simulink model "bluetooth_voice"  (Simulink 6.0)
settings: Solver=ode3  SolverMode=SingleTasking  StartTime=0.0  StopTime=2.7  RelTol=1e-3
PreLoadFcn:
  | bluetooth_init;
PostLoadFcn:
  | bluetooth_cb
values from neighbouring files (symbols this model uses):
  Access_Code = zeros(72,1); Access_Code(1:2:72)=1    [bluetooth_init.m]
  ARQ = [1]    [bluetooth_init.m]
  awgn_802_seed = randseed(3)    [bluetooth_init.m]
  awgn_channel_seed = randseed(2)    [bluetooth_init.m]
  data_seed = randseed(5)    [bluetooth_init.m]
  Flow_Control = [1]    [bluetooth_init.m]
  HV_Type = 3    [bluetooth_cb.m]
  Input_Fs = 8000    [bluetooth_init.m]
  One_Zero_Payload = zeros(240,1)    [bluetooth_init.m]
  Packet_Type = [1 0 1 0]'    [bluetooth_init.m]
  rate_802_seed = randseed(4)    [bluetooth_init.m]
  Sequence = [1]    [bluetooth_init.m]
  Slave_Address = [1 0 1]'    [bluetooth_init.m]
  Slot_Ts = (1/1600)    (= 0.000625)    [bluetooth_cb.m]
undefined symbols (not defined in the file or in its folder): figposition, Fs, jet, Num_Slots_Rate, slcm, Slot_Enable_Phase, Tx_Ts
libraries: commblkcod2 x48, dspsrcs4 x22, dspsigops x19, simulink x15, dspbuff3 x8, dspindex x7, dspsigattribs x6, dspmtrx3 x5, dsparch4 x4, commdigbbndfm2 x4, bluetooth_lib x4, dspsnks4 x4
(part 2 of 2)

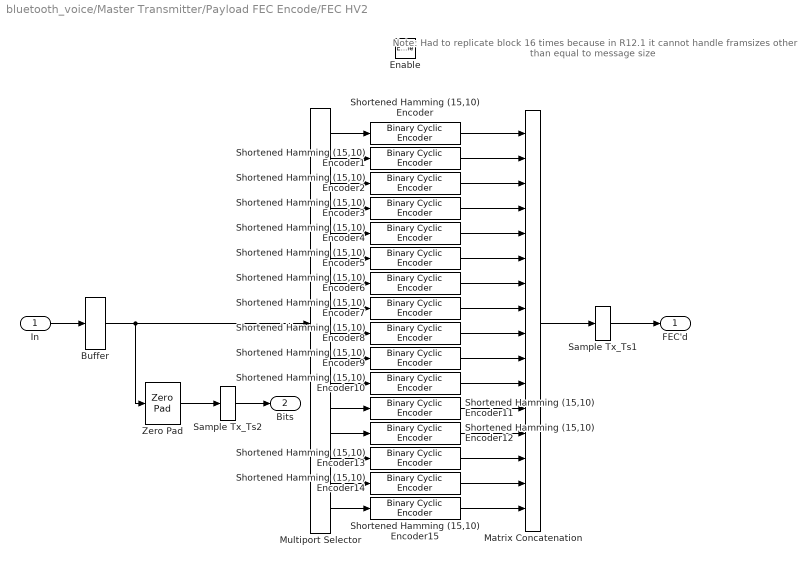
== system bluetooth_voice/Master Transmitter/Payload FEC Encode/FEC HV2 ==
  note: Note: Had to replicate block 16 times
      | because in R12.1 it cannot handle framsizes
      | other than equal to message size
  In : Inport  LatchInput=off
  Enable : EnablePort
  Buffer : dspbuff3/Buffer  N=160  V=0  ic=0
  Matrix Concatenation : simulink/Math Operations/Matrix Concatenation  numInports=16  catMethod=Vertical
  Multiport Selector : dspindex/Multiport Selector  rowsOrCols=Rows  idxCellArray={ 1:10, 11:20,21:30,31:40,41:50,51:60,61:70,71:80,81:90,91:100,101:110,111:120,121:130,131:140,141:150,151:160}  idxErrMode=Clip Index
  Sample Tx_Ts1 : ZeroOrderHold  SampleTime=Slot_Ts
  Sample Tx_Ts2 : ZeroOrderHold  SampleTime=Slot_Ts
  Shortened Hamming (15,10) Encoder{,1..15} (16 alike) : commblkcod2/Binary Cyclic Encoder  n=15  p=[1 1 0 1 0 1]
  Zero Pad : dspsigops/Zero Pad  padSigAt=End  zpadAlong=Columns  padNumOutRowsSpecMethod=User-specified  numOutRows=240  padNumOutColsSpecMethod=User-specified  numOutCols=1  trunc_flag=None
  FEC'd : Outport
  Bits : Outport  Port=2
  wires:
  In/1 -> Buffer/1
  Buffer/1 -> Multiport Selector/1, Zero Pad/1
  Multiport Selector/1 -> Shortened Hamming (15,10) Encoder/1
  Multiport Selector/2 -> Shortened Hamming (15,10) Encoder1/1
  Multiport Selector/3 -> Shortened Hamming (15,10) Encoder2/1
  Multiport Selector/4 -> Shortened Hamming (15,10) Encoder3/1
  Multiport Selector/5 -> Shortened Hamming (15,10) Encoder4/1
  Multiport Selector/6 -> Shortened Hamming (15,10) Encoder5/1
  Multiport Selector/7 -> Shortened Hamming (15,10) Encoder6/1
  Multiport Selector/8 -> Shortened Hamming (15,10) Encoder7/1
  Multiport Selector/9 -> Shortened Hamming (15,10) Encoder8/1
  Multiport Selector/10 -> Shortened Hamming (15,10) Encoder9/1
  Multiport Selector/11 -> Shortened Hamming (15,10) Encoder10/1
  Multiport Selector/12 -> Shortened Hamming (15,10) Encoder11/1
  Multiport Selector/13 -> Shortened Hamming (15,10) Encoder12/1
  Multiport Selector/14 -> Shortened Hamming (15,10) Encoder13/1
  Multiport Selector/15 -> Shortened Hamming (15,10) Encoder14/1
  Multiport Selector/16 -> Shortened Hamming (15,10) Encoder15/1
  Shortened Hamming (15,10) Encoder/1 -> Matrix Concatenation/1
  Shortened Hamming (15,10) Encoder1/1 -> Matrix Concatenation/2
  Shortened Hamming (15,10) Encoder2/1 -> Matrix Concatenation/3
  Shortened Hamming (15,10) Encoder3/1 -> Matrix Concatenation/4
  Shortened Hamming (15,10) Encoder4/1 -> Matrix Concatenation/5
  Shortened Hamming (15,10) Encoder5/1 -> Matrix Concatenation/6
  Shortened Hamming (15,10) Encoder6/1 -> Matrix Concatenation/7
  Shortened Hamming (15,10) Encoder7/1 -> Matrix Concatenation/8
  Shortened Hamming (15,10) Encoder8/1 -> Matrix Concatenation/9
  Shortened Hamming (15,10) Encoder9/1 -> Matrix Concatenation/10
  Shortened Hamming (15,10) Encoder10/1 -> Matrix Concatenation/11
  Shortened Hamming (15,10) Encoder11/1 -> Matrix Concatenation/12
  Shortened Hamming (15,10) Encoder12/1 -> Matrix Concatenation/13
  Shortened Hamming (15,10) Encoder13/1 -> Matrix Concatenation/14
  Shortened Hamming (15,10) Encoder14/1 -> Matrix Concatenation/15
  Shortened Hamming (15,10) Encoder15/1 -> Matrix Concatenation/16
  Matrix Concatenation/1 -> Sample Tx_Ts1/1
  Zero Pad/1 -> Sample Tx_Ts2/1
  Sample Tx_Ts1/1 -> FEC'd/1
  Sample Tx_Ts2/1 -> Bits/1

== system bluetooth_voice/Master Transmitter/Payload FEC Encode/FEC HV3 (None) ==
  In : Inport  LatchInput=off
  Enable : EnablePort
  Buffer : dspbuff3/Buffer  N=240  V=0  ic=0
  Sample Tx_Ts1 : ZeroOrderHold  SampleTime=Slot_Ts
  Sample Tx_Ts2 : ZeroOrderHold  SampleTime=Slot_Ts
  FEC'd : Outport
  Bits : Outport  Port=2
  wires:
  In/1 -> Buffer/1
  Sample Tx_Ts1/1 -> FEC'd/1
  Sample Tx_Ts2/1 -> Bits/1
  Buffer/1 -> Sample Tx_Ts1/1, Sample Tx_Ts2/1

== system bluetooth_voice/Scopes/Subsystem/Marker ==
  Enable : EnablePort
  DSP Constant : dspsrcs4/DSP Constant  Value=.1*[ones(1,36600) zeros(1,62500-36600)]'  SampleMode=Discrete  discreteOutput=Frame-based  continuousOutput=Sample-based  sampTime=625e-6  framePeriod=625e-6  dataType=Inherit from 'Constant value'  isSigned=on  wordLen=16  udDataType=sfix(16)  fracBitsMode=Best precision  numFracBits=15  InterpretAs1D=off  Ts=625e-6  FramebasedOutput=on
  Tx : Outport  OutputWhenDisabled=reset  InitialOutput=0
  wires:
  DSP Constant/1 -> Tx/1

== system bluetooth_voice/Slave Receiver/CVSD Decode/Update accum ==
  stepsize(n+1) : Inport  LatchInput=off
  u : Inport  Port=2  LatchInput=off
  accum(n) : Inport  Port=3  LatchInput=off
  Gain : Gain  Gain=accum_decay  SaturateOnIntegerOverflow=on
  Product : Product  SaturateOnIntegerOverflow=on  InputSameDT=on
  Saturation : Saturate  UpperLimit=pos_accum_max  LowerLimit=neg_accum_max
  Sum1 : Sum  Inputs=|++  SaturateOnIntegerOverflow=on  InputSameDT=on
  accum(n+1) : Outport
  wires:
  Product/1 -> Sum1/1  "y*stepsize"
  Sum1/1 -> Gain/1
  stepsize(n+1)/1 -> Product/1
  u/1 -> Product/2
  accum(n)/1 -> Sum1/2
  Gain/1 -> Saturation/1
  Saturation/1 -> accum(n+1)/1

== system bluetooth_voice/Slave Receiver/CVSD Decode/Update runner ==
  u : Inport  LatchInput=off
  runner(n) : Inport  Port=2  LatchInput=off
  Bitwise Logical Operator : simulink/Logic and Bit Operations/Bitwise Operator  logicop=AND  UseBitMask=on  BitMask=15  BitMaskRealWorld=Stored Integer
  Data Type Conversion : DataTypeConversion  OutDataTypeMode=uint16  SaturateOnIntegerOverflow=on  RndMeth=Zero
  Data Type Conversion1 : DataTypeConversion  OutDataTypeMode=double  SaturateOnIntegerOverflow=on  RndMeth=Zero
  Fcn : Fcn  Expr=u==1
  Gain : Gain  Gain=2  SaturateOnIntegerOverflow=on
  Sum1 : Sum  Inputs=|++  SaturateOnIntegerOverflow=on  InputSameDT=on
  runner(n+1) : Outport
  wires:
  Gain/1 -> Sum1/2  "2*runner"
  Fcn/1 -> Sum1/1  "y==1"
  Sum1/1 -> Data Type Conversion/1
  Data Type Conversion/1 -> Bitwise Logical Operator/1
  u/1 -> Fcn/1
  Bitwise Logical Operator/1 -> Data Type Conversion1/1
  runner(n)/1 -> Gain/1
  Data Type Conversion1/1 -> runner(n+1)/1

== system bluetooth_voice/Slave Receiver/CVSD Decode/Update stepsize ==
  runner(n+1) : Inport  LatchInput=off
  stepsize(n) : Inport  Port=2  LatchInput=off
  If : If  IfExpression=(u1 == 0) | (u1== 15)
  Merge1 : Merge
  Update : Subsystem  TreatAsAtomicUnit=on  PropExecContextAcrossSSBoundary=on
  Update1 : Subsystem  TreatAsAtomicUnit=on  PropExecContextAcrossSSBoundary=on
  stepsize(n+1) : Outport
  wires:
  If/1 -> Update/Action  "(runner == 0) | (runner == 15)"
  Update/1(stepsize(n+1)) -> Merge1/1
  stepsize(n)/1 -> Update1/1(stepsize), Update/1(stepsize)
  If/2 -> Update1/Action
  Update1/1(stepsize(n+1)) -> Merge1/2
  runner(n+1)/1 -> If/1
  Merge1/1 -> stepsize(n+1)/1

== system bluetooth_voice/Slave Receiver/Demodulate and decode/Access Code Fail ==
  In : Inport  LatchInput=off
  Access Code : dspsrcs4/DSP Constant  Value=Access_Code  SampleMode=Discrete  discreteOutput=Frame-based  continuousOutput=Sample-based  sampTime=Slot_Ts  framePeriod=Slot_Ts  dataType=Inherit from 'Constant value'  isSigned=on  wordLen=16  udDataType=sfix(16)  fracBitsMode=Best precision  numFracBits=15  InterpretAs1D=off  Ts=Slot_Ts  FramebasedOutput=on
  Constant : Constant  Value=57
  Less than  57 bits good : RelationalOperator  Operator=<  InputSameDT=on
  Relational Operator : RelationalOperator  Operator===  InputSameDT=on
  Strip of preamble  and trailer : Selector  Elements=[5:68]  InputPortWidth=72
  Strip of preamble  and trailer1 : Selector  Elements=[5:68]  InputPortWidth=72
  Total correct bits : Sum  Inputs=1  SaturateOnIntegerOverflow=on  InputSameDT=on
  Out : Outport
  wires:
  Less than  57 bits good/1 -> Out/1
  In/1 -> Strip of preamble  and trailer1/1
  Constant/1 -> Less than  57 bits good/2
  Total correct bits/1 -> Less than  57 bits good/1
  Strip of preamble  and trailer/1 -> Relational Operator/1
  Strip of preamble  and trailer1/1 -> Relational Operator/2
  Relational Operator/1 -> Total correct bits/1
  Access Code/1 -> Strip of preamble  and trailer/1

== system bluetooth_voice/Slave Receiver/Demodulate and decode/GMSK Demodulate and frequency hop ==
  Rx Signal : Inport  LatchInput=off
  Hop : Inport  Port=2  LatchInput=off
  Extract 366 bits with one symbol delay : Selector  Elements=[2:367]  InputPortWidth=625
  Frame Status Conversion : dspsigattribs/Frame Status Conversion  growRefPort=off  outframe=Frame-based
  "Generate 79 possible carriers -39MHz to 39MHz " : commdigbbndfm2/M-FSK Modulator Baseband  M=79  InType=Integer  Enc=Binary  freqSep=1e6  phaseType=Continuous  numSamp=6.25e4
  IF Filter Select 1MHz band1 : dsparch4/Digital Filter Design
  M-FSK Demodulator Baseband : commdigbbndfm2/M-FSK Demodulator Baseband  M=2  OutType=Bit  Dec=Binary  freqSep=2*150e3  numSamp=100
  Math Function : Math  Orientation=up  Operator=conj  SaturateOnIntegerOverflow=on
  Move to a symbol boundary : dspsigops/Delay  dly_unit=Samples  delay=100-50  ic_detail=off  dif_ic_for_ch=off  dif_ic_for_dly=off  ic=0  reset_popup=None
  Product1 : Product  SaturateOnIntegerOverflow=on  InputSameDT=on
  Rx Raw Bits : Outport
  wires:
  Move to a symbol boundary/1 -> M-FSK Demodulator Baseband/1
  Frame Status Conversion/1 -> "Generate 79 possible carriers -39MHz to 39MHz "/1
  "Generate 79 possible carriers -39MHz to 39MHz "/1 -> Math Function/1
  Math Function/1 -> Product1/2
  Product1/1 -> IF Filter Select 1MHz band1/1
  M-FSK Demodulator Baseband/1 -> Extract 366 bits with one symbol delay/1
  Rx Signal/1 -> Product1/1
  Extract 366 bits with one symbol delay/1 -> Rx Raw Bits/1
  Hop/1 -> Frame Status Conversion/1
  IF Filter Select 1MHz band1/1 -> Move to a symbol boundary/1

== system bluetooth_voice/Slave Receiver/Demodulate and decode/HEC Fail ==
  In : Inport  LatchInput=off
  General CRC Syndrome Detector : commcrc2/General CRC Syndrome Detector  genPoly=[1 1 0 1 0 0 1 1 1]  iniStates=[1 0 0 1 0 1 1 0]  numChecksums=1
  Terminator : Terminator
  Out : Outport
  wires:
  In/1 -> General CRC Syndrome Detector/1
  General CRC Syndrome Detector/2 -> Out/1
  General CRC Syndrome Detector/1 -> Terminator/1

== system bluetooth_voice/Slave Receiver/Demodulate and decode/Header info FEC Decode ==
  In : Inport  LatchInput=off
  Constant1 : Constant  Value=.5
  Decode FEC : commsequence2/Derepeat  N=3  ic=0  mode=Maintain input frame rate
  Threshold : RelationalOperator  Operator=>  InputSameDT=on
  Out : Outport
  wires:
  Threshold/1 -> Out/1  "HEC"
  In/1 -> Decode FEC/1
  Decode FEC/1 -> Threshold/1
  Constant1/1 -> Threshold/2

== system bluetooth_voice/Slave Receiver/Demodulate and decode/One Zeros ==
  Constant : Constant  Value=HV_Type
  FEC HV1 : Subsystem  TreatAsAtomicUnit=on  PropExecContextAcrossSSBoundary=on
  FEC HV2 : Subsystem  TreatAsAtomicUnit=on  PropExecContextAcrossSSBoundary=on
  FEC HV3 (None) : Subsystem  TreatAsAtomicUnit=on  PropExecContextAcrossSSBoundary=on
  Fcn : Fcn  Expr=u==1
  Fcn1 : Fcn  Expr=u==2
  Fcn2 : Fcn  Expr=u==3
  Merge : Merge  Inputs=3
  One Zeros : Outport
  wires:
  Constant/1 -> Fcn/1, Fcn1/1, Fcn2/1
  Fcn/1 -> FEC HV1/Enable
  Fcn1/1 -> FEC HV2/Enable
  Fcn2/1 -> FEC HV3 (None)/Enable
  FEC HV2/1(Ones Zeros) -> Merge/2
  FEC HV1/1(Ones Zeros) -> Merge/1
  Merge/1 -> One Zeros/1
  FEC HV3 (None)/1(Ones Zeros) -> Merge/3

== system bluetooth_voice/Slave Receiver/Demodulate and decode/Payload FEC Decode ==
  Input Bits : Inport  LatchInput=off
  Constant : Constant  Value=HV_Type
  FEC HV1 : Subsystem  TreatAsAtomicUnit=on  PropExecContextAcrossSSBoundary=on
  FEC HV2 : Subsystem  TreatAsAtomicUnit=on  PropExecContextAcrossSSBoundary=on
  FEC HV3 (None) : Subsystem  TreatAsAtomicUnit=on  PropExecContextAcrossSSBoundary=on
  Fcn : Fcn  Expr=u==1
  Fcn1 : Fcn  Expr=u==2
  Fcn2 : Fcn  Expr=u==3
  Merge : Merge  Inputs=3
  Payload Bits1 : dspindex/Multiport Selector  rowsOrCols=Rows  idxCellArray={1:Num_Payload_Bits}  idxErrMode=Clip Index
  Decoded Bits : Outport
  wires:
  Payload Bits1/1 -> Decoded Bits/1
  Merge/1 -> Payload Bits1/1
  FEC HV3 (None)/1(FEC'd) -> Merge/3
  FEC HV1/1(FEC'd) -> Merge/1
  FEC HV2/1(FEC'd) -> Merge/2
  Fcn2/1 -> FEC HV3 (None)/Enable
  Fcn1/1 -> FEC HV2/Enable
  Fcn/1 -> FEC HV1/Enable
  Constant/1 -> Fcn1/1, Fcn2/1, Fcn/1
  Input Bits/1 -> FEC HV1/1(In), FEC HV2/1(In), FEC HV3 (None)/1(In)

== system bluetooth_voice/Slave Receiver/Demodulate and decode/Residual BER Subsystem ==
  In1 : Inport  LatchInput=off
  In2 : Inport  Port=2  LatchInput=off
  Enable : EnablePort
  Residual BER : commsink2/Error Rate Calculation  N=0  st_delay=0  cp_mode=Entire frame  subframe=[]  PMode=Port  WsName=ErrorVec  RsMode2=off  stop=off  numErr=100  maxBits=1e6
  Out1 : Outport
  wires:
  In2/1 -> Residual BER/2
  Residual BER/1 -> Out1/1
  In1/1 -> Residual BER/1

== system bluetooth_voice/Master Transmitter/CVSD Encode/Set any 0's to 1's/Pass through ==
  In1 : Inport  LatchInput=off
  Action Port : ActionPort  ActionType=else
  Out1=In1 : Outport
  wires:
  In1/1 -> Out1=In1/1

== system bluetooth_voice/Master Transmitter/CVSD Encode/Set any 0's to 1's/Set to 1 ==
  Action Port : ActionPort  ActionType=then
  DSP Constant : dspsrcs4/DSP Constant  Value=1  SampleMode=Discrete  discreteOutput=Sample-based (interpret vectors as 1-D)  continuousOutput=Sample-based (interpret vectors as 1-D)  sampTime=1/64000  framePeriod=1/64000  dataType=Inherit from 'Constant value'  isSigned=on  wordLen=16  udDataType=sfix(16)  fracBitsMode=Best precision  numFracBits=15  InterpretAs1D=on  Ts=1/64000  FramebasedOutput=off
  1 : Outport  InitialOutput=1
  wires:
  DSP Constant/1 -> 1/1

== system bluetooth_voice/Master Transmitter/CVSD Encode/Update stepsize/Update ==
  stepsize : Inport  LatchInput=off
  Action Port : ActionPort  ActionType=then
  Constant : Constant  Value=min_step
  Constant1 : Constant  Value=max_step
  MinMax : MinMax  Inputs=2  SaturateOnIntegerOverflow=on  InputSameDT=on
  Sum2 : Sum  Inputs=|++  SaturateOnIntegerOverflow=on  InputSameDT=on
  stepsize(n+1) : Outport
  wires:
  Constant/1 -> Sum2/1
  Sum2/1 -> MinMax/1
  Constant1/1 -> MinMax/2
  MinMax/1 -> stepsize(n+1)/1
  stepsize/1 -> Sum2/2

== system bluetooth_voice/Master Transmitter/CVSD Encode/Update stepsize/Update1 ==
  stepsize : Inport  LatchInput=off
  Action Port : ActionPort  ActionType=else
  Constant1 : Constant  Value=min_step
  Gain : Gain  Gain=step_decay  SaturateOnIntegerOverflow=on
  MinMax : MinMax  Function=max  Inputs=2  SaturateOnIntegerOverflow=on  InputSameDT=on
  stepsize(n+1) : Outport
  wires:
  MinMax/1 -> stepsize(n+1)/1
  Constant1/1 -> MinMax/2
  Gain/1 -> MinMax/1
  stepsize/1 -> Gain/1

== system bluetooth_voice/Slave Receiver/CVSD Decode/Update stepsize/Update ==
  stepsize : Inport  LatchInput=off
  Action Port : ActionPort  ActionType=then
  Constant : Constant  Value=min_step
  Constant1 : Constant  Value=max_step
  MinMax : MinMax  Inputs=2  SaturateOnIntegerOverflow=on  InputSameDT=on
  Sum2 : Sum  Inputs=|++  SaturateOnIntegerOverflow=on  InputSameDT=on
  stepsize(n+1) : Outport
  wires:
  Constant/1 -> Sum2/1
  Sum2/1 -> MinMax/1
  Constant1/1 -> MinMax/2
  MinMax/1 -> stepsize(n+1)/1
  stepsize/1 -> Sum2/2

== system bluetooth_voice/Slave Receiver/CVSD Decode/Update stepsize/Update1 ==
  stepsize : Inport  LatchInput=off
  Action Port : ActionPort  ActionType=else
  Constant1 : Constant  Value=min_step
  Gain : Gain  Gain=step_decay  SaturateOnIntegerOverflow=on
  MinMax : MinMax  Function=max  Inputs=2  SaturateOnIntegerOverflow=on  InputSameDT=on
  stepsize(n+1) : Outport
  wires:
  MinMax/1 -> stepsize(n+1)/1
  Constant1/1 -> MinMax/2
  Gain/1 -> MinMax/1
  stepsize/1 -> Gain/1

== system bluetooth_voice/Slave Receiver/Demodulate and decode/One Zeros/FEC HV1 ==
  Enable : EnablePort
  1 0 1 0 1 0 ... : dspsrcs4/DSP Constant  Value=One_Zero_Payload(1:80)  SampleMode=Discrete  discreteOutput=Frame-based  continuousOutput=Sample-based  sampTime=30*(1/Input_Fs)/6  framePeriod=30*(1/Input_Fs)/6  dataType=Inherit from 'Constant value'  isSigned=on  wordLen=16  udDataType=sfix(16)  fracBitsMode=Best precision  numFracBits=15  InterpretAs1D=off  Ts=30*(1/Input_Fs)/6  FramebasedOutput=on
  FEC1 : dspsigops/Repeat  N=3  ic=0  mode=Maintain input frame rate
  Ones Zeros : Outport
  wires:
  1 0 1 0 1 0 .../1 -> FEC1/1
  FEC1/1 -> Ones Zeros/1

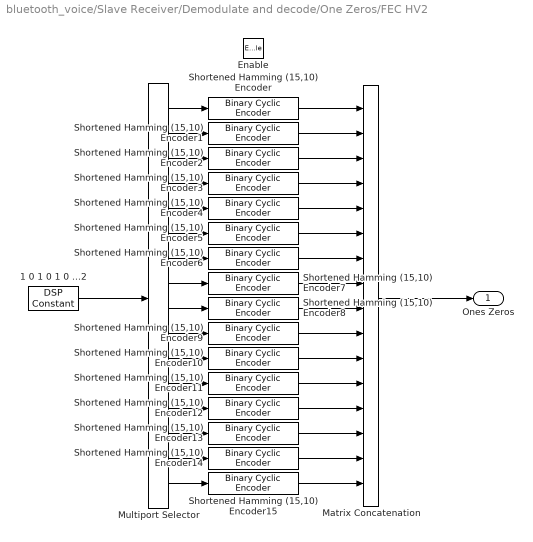
== system bluetooth_voice/Slave Receiver/Demodulate and decode/One Zeros/FEC HV2 ==
  Enable : EnablePort
  1 0 1 0 1 0 ...2 : dspsrcs4/DSP Constant  Value=One_Zero_Payload(1:160)  SampleMode=Discrete  discreteOutput=Frame-based  continuousOutput=Sample-based  sampTime=Slot_Ts  framePeriod=Slot_Ts  dataType=Inherit from 'Constant value'  isSigned=on  wordLen=16  udDataType=sfix(16)  fracBitsMode=Best precision  numFracBits=15  InterpretAs1D=off  Ts=Slot_Ts  FramebasedOutput=on
  Matrix Concatenation : simulink/Math Operations/Matrix Concatenation  numInports=16  catMethod=Vertical
  Multiport Selector : dspindex/Multiport Selector  rowsOrCols=Rows  idxCellArray={ 1:10, 11:20,21:30,31:40,41:50,51:60,61:70,71:80,81:90,91:100,101:110,111:120,121:130,131:140,141:150,151:160}  idxErrMode=Clip Index
  Shortened Hamming (15,10) Encoder{,1..15} (16 alike) : commblkcod2/Binary Cyclic Encoder  n=15  p=[1 1 0 1 0 1]
  Ones Zeros : Outport
  wires:
  1 0 1 0 1 0 ...2/1 -> Multiport Selector/1
  Multiport Selector/1 -> Shortened Hamming (15,10) Encoder/1
  Multiport Selector/2 -> Shortened Hamming (15,10) Encoder1/1
  Multiport Selector/3 -> Shortened Hamming (15,10) Encoder2/1
  Multiport Selector/4 -> Shortened Hamming (15,10) Encoder3/1
  Multiport Selector/5 -> Shortened Hamming (15,10) Encoder4/1
  Multiport Selector/6 -> Shortened Hamming (15,10) Encoder5/1
  Multiport Selector/7 -> Shortened Hamming (15,10) Encoder6/1
  Multiport Selector/8 -> Shortened Hamming (15,10) Encoder7/1
  Multiport Selector/9 -> Shortened Hamming (15,10) Encoder8/1
  Multiport Selector/10 -> Shortened Hamming (15,10) Encoder9/1
  Multiport Selector/11 -> Shortened Hamming (15,10) Encoder10/1
  Multiport Selector/12 -> Shortened Hamming (15,10) Encoder11/1
  Multiport Selector/13 -> Shortened Hamming (15,10) Encoder12/1
  Multiport Selector/14 -> Shortened Hamming (15,10) Encoder13/1
  Multiport Selector/15 -> Shortened Hamming (15,10) Encoder14/1
  Multiport Selector/16 -> Shortened Hamming (15,10) Encoder15/1
  Shortened Hamming (15,10) Encoder/1 -> Matrix Concatenation/1
  Shortened Hamming (15,10) Encoder1/1 -> Matrix Concatenation/2
  Shortened Hamming (15,10) Encoder2/1 -> Matrix Concatenation/3
  Shortened Hamming (15,10) Encoder3/1 -> Matrix Concatenation/4
  Shortened Hamming (15,10) Encoder4/1 -> Matrix Concatenation/5
  Shortened Hamming (15,10) Encoder5/1 -> Matrix Concatenation/6
  Shortened Hamming (15,10) Encoder6/1 -> Matrix Concatenation/7
  Shortened Hamming (15,10) Encoder7/1 -> Matrix Concatenation/8
  Shortened Hamming (15,10) Encoder8/1 -> Matrix Concatenation/9
  Shortened Hamming (15,10) Encoder9/1 -> Matrix Concatenation/10
  Shortened Hamming (15,10) Encoder10/1 -> Matrix Concatenation/11
  Shortened Hamming (15,10) Encoder11/1 -> Matrix Concatenation/12
  Shortened Hamming (15,10) Encoder12/1 -> Matrix Concatenation/13
  Shortened Hamming (15,10) Encoder13/1 -> Matrix Concatenation/14
  Shortened Hamming (15,10) Encoder14/1 -> Matrix Concatenation/15
  Shortened Hamming (15,10) Encoder15/1 -> Matrix Concatenation/16
  Matrix Concatenation/1 -> Ones Zeros/1

== system bluetooth_voice/Slave Receiver/Demodulate and decode/One Zeros/FEC HV3 (None) ==
  Enable : EnablePort
  1 0 1 0 1 0 ... : dspsrcs4/DSP Constant  Value=One_Zero_Payload(1:240)  SampleMode=Discrete  discreteOutput=Frame-based  continuousOutput=Sample-based  sampTime=1/1600  framePeriod=1/1600  dataType=Inherit from 'Constant value'  isSigned=on  wordLen=16  udDataType=sfix(16)  fracBitsMode=Best precision  numFracBits=15  InterpretAs1D=off  Ts=1/1600  FramebasedOutput=on
  Ones Zeros : Outport  InitialOutput=One_Zero_Payload(1:240)
  wires:
  1 0 1 0 1 0 .../1 -> Ones Zeros/1

== system bluetooth_voice/Slave Receiver/Demodulate and decode/Payload FEC Decode/FEC HV1 ==
  In : Inport  LatchInput=off
  Enable : EnablePort
  Constant1 : Constant  Value=.5
  Decode FEC : commsequence2/Derepeat  N=3  ic=One_Zero_Payload(1:80)  mode=Maintain input frame rate
  Threshold : RelationalOperator  Operator=>  InputSameDT=on
  Zero Pad : dspsigops/Zero Pad  padSigAt=End  zpadAlong=Columns  padNumOutRowsSpecMethod=User-specified  numOutRows=240  padNumOutColsSpecMethod=User-specified  numOutCols=1  trunc_flag=None
  FEC'd : Outport
  wires:
  Zero Pad/1 -> FEC'd/1
  Decode FEC/1 -> Threshold/1
  Constant1/1 -> Threshold/2
  Threshold/1 -> Zero Pad/1
  In/1 -> Decode FEC/1

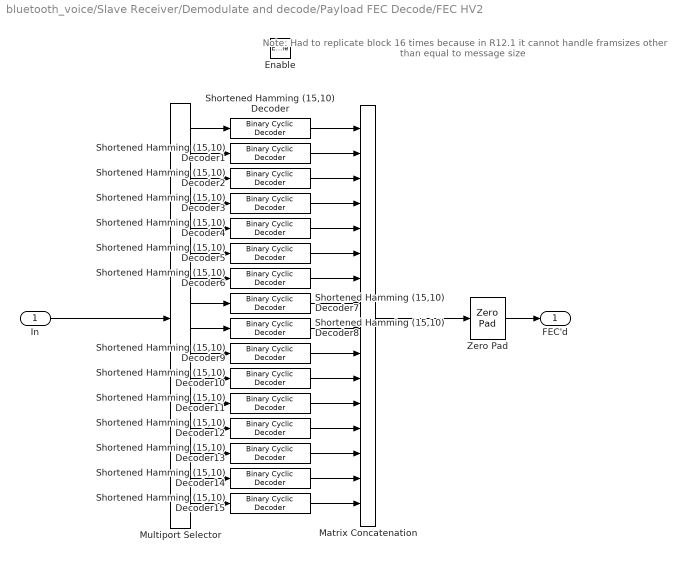
== system bluetooth_voice/Slave Receiver/Demodulate and decode/Payload FEC Decode/FEC HV2 ==
  note: Note: Had to replicate block 16 times
      | because in R12.1 it cannot handle framsizes
      | other than equal to message size
  In : Inport  LatchInput=off
  Enable : EnablePort
  Matrix Concatenation : simulink/Math Operations/Matrix Concatenation  numInports=16  catMethod=Vertical
  Multiport Selector : dspindex/Multiport Selector  rowsOrCols=Rows  idxCellArray={ 1:15, 16:30,31:45,46:60,61:75,76:90,91:105,106:120,121:135,136:150,151:165,166:180,181:195,196:210,211:225,226:240}  idxErrMode=Clip Index
  Shortened Hamming (15,10) Decoder{,1..15} (16 alike) : commblkcod2/Binary Cyclic Decoder  n=15  p=[1 1 0 1 0 1]
  Zero Pad : dspsigops/Zero Pad  padSigAt=End  zpadAlong=Columns  padNumOutRowsSpecMethod=User-specified  numOutRows=240  padNumOutColsSpecMethod=User-specified  numOutCols=1  trunc_flag=None
  FEC'd : Outport
  wires:
  Zero Pad/1 -> FEC'd/1
  Shortened Hamming (15,10) Decoder15/1 -> Matrix Concatenation/16
  Shortened Hamming (15,10) Decoder14/1 -> Matrix Concatenation/15
  Shortened Hamming (15,10) Decoder13/1 -> Matrix Concatenation/14
  Shortened Hamming (15,10) Decoder12/1 -> Matrix Concatenation/13
  Shortened Hamming (15,10) Decoder11/1 -> Matrix Concatenation/12
  Shortened Hamming (15,10) Decoder10/1 -> Matrix Concatenation/11
  Shortened Hamming (15,10) Decoder9/1 -> Matrix Concatenation/10
  Shortened Hamming (15,10) Decoder8/1 -> Matrix Concatenation/9
  Shortened Hamming (15,10) Decoder7/1 -> Matrix Concatenation/8
  Shortened Hamming (15,10) Decoder6/1 -> Matrix Concatenation/7
  Shortened Hamming (15,10) Decoder5/1 -> Matrix Concatenation/6
  Shortened Hamming (15,10) Decoder4/1 -> Matrix Concatenation/5
  Shortened Hamming (15,10) Decoder3/1 -> Matrix Concatenation/4
  Shortened Hamming (15,10) Decoder2/1 -> Matrix Concatenation/3
  Shortened Hamming (15,10) Decoder1/1 -> Matrix Concatenation/2
  Shortened Hamming (15,10) Decoder/1 -> Matrix Concatenation/1
  Matrix Concatenation/1 -> Zero Pad/1
  Multiport Selector/16 -> Shortened Hamming (15,10) Decoder15/1
  Multiport Selector/15 -> Shortened Hamming (15,10) Decoder14/1
  Multiport Selector/14 -> Shortened Hamming (15,10) Decoder13/1
  Multiport Selector/13 -> Shortened Hamming (15,10) Decoder12/1
  Multiport Selector/12 -> Shortened Hamming (15,10) Decoder11/1
  Multiport Selector/11 -> Shortened Hamming (15,10) Decoder10/1
  Multiport Selector/10 -> Shortened Hamming (15,10) Decoder9/1
  Multiport Selector/9 -> Shortened Hamming (15,10) Decoder8/1
  Multiport Selector/8 -> Shortened Hamming (15,10) Decoder7/1
  Multiport Selector/7 -> Shortened Hamming (15,10) Decoder6/1
  Multiport Selector/6 -> Shortened Hamming (15,10) Decoder5/1
  Multiport Selector/5 -> Shortened Hamming (15,10) Decoder4/1
  Multiport Selector/4 -> Shortened Hamming (15,10) Decoder3/1
  Multiport Selector/3 -> Shortened Hamming (15,10) Decoder2/1
  Multiport Selector/2 -> Shortened Hamming (15,10) Decoder1/1
  Multiport Selector/1 -> Shortened Hamming (15,10) Decoder/1
  In/1 -> Multiport Selector/1

== system bluetooth_voice/Slave Receiver/Demodulate and decode/Payload FEC Decode/FEC HV3 (None) ==
  In : Inport  LatchInput=off
  Enable : EnablePort
  FEC'd : Outport
  wires:
  In/1 -> FEC'd/1
